simulink model "StandaloneDAQv07_R2014a"  (R2014a)
settings: Solver=FixedStepDiscrete  SolverMode=MultiTasking  StartTime=0.0  StopTime=inf  FixedStep=0.0005  RelTol=1e-3
values from neighbouring files (symbols this model uses):
  ANOMALY_INIT = 10    [DAQParams3_1ms_DDA.m]
  Calibration = getCalibrationParams_ATRIAS()    [DAQParams3_1ms_DDA.m]
  EnableFT = 0    [DAQParams3_1ms_DDA.m]
  EncoderAngleLimits = [60 240; 120 300; 60 240; 120 300; 60 240; 120 300; 60 240; 120 300; -30 30; -30 30; -inf inf; -inf inf; -inf inf; -inf inf; -30 30; -30 30; -inf inf; -90 90; -90 90]*pi/180    [DAQParams3_1ms_DDA.m]
  EncoderFiltSys = getDerivFilter(2, 5, 5, Ts)    [DAQParams3_1ms_DDA.m]
  EncoderThreshold = [5; 5; 5; 5; 5; 5; 5; 5; 5; 5; 250; 250; 250; 250; 5; 5; 5; 5; 5]*pi/180    [DAQParams3_1ms_DDA.m]
  IMUAngleLimits = [-180 180; -90 90; -90 90]*pi/180    [DAQParams3_1ms_DDA.m]
  IMUCommand = 70    [DAQParams3_1ms_DDA.m]
  IMUThreshold = 5*pi/180    (= 0.0872664625997)    [DAQParams3_1ms_DDA.m]
  MAX_ANOMALY = 30    [DAQParams3_1ms_DDA.m]
  MedullaCommand = 0    [DAQParams3_1ms_DDA.m]
  MicrostrainFiltSys = getDerivFilter(2, 5, 5, TsMicrostrain)    [DAQParams3_1ms_DDA.m]
  MODBUS_TIMEOUT = 0.02    [DAQParams3_1ms_DDA.m]
  ResetDAQ = 0    [DAQParams3_1ms_DDA.m]
  ResetYaw = 0    [DAQParams3_1ms_DDA.m]
  STREAMING_TIMEOUT = 0.1    [DAQParams3_1ms_DDA.m]
  TareFT = 0    [DAQParams3_1ms_DDA.m]
  Ts = 0.001    [DAQParams3_1ms_DDA.m]
  UseMicrostrainRate = 0    [DAQParams3_1ms_DDA.m]
undefined symbols (not defined in the file or in its folder): FTCalibration, GearOffset, IMUTorsoOffset, m_XR17D15x, standard
libraries: xpcethercatlib x167, speedgoatlib x13, dspswit3 x2, simulink x2, xpcseriallib x1, SpeedgoatModified x1
(part 4 of 4)

== matlab function StandaloneDAQv07_R2014a/SerialInterfaces/FTInterface/Subsystem/ComputeCalibratedTorques/ComputeCalibratedTorques ==
  data: Gauge input; FT output; Bias input; Cal input
function FT = fcn(Gauge, Bias, Cal)
    %#codegen
    FT = Cal.BasicMatrix * (Gauge - Bias);
    FT(1:3,:) = FT(1:3,:) / Cal.CountsPerForce;
    FT(4:6,:) = FT(4:6,:) / Cal.CountsPerTorque;
end

== stateflow chart StandaloneDAQv07_R2014a/EtherCATNetwork/EncoderFilters/CheckAndFilterEncoder/AnomalyDetection ==
  state Run
    state Nominal
      en, du:
      q_clean = q;
      q_last = q;
      dq_last = dq;
      Counter_last = Counter;
      ErrorCount = 0;
    state MissedPacket
      en, du:
      q_clean = q_last + dq_last*ANOMALY_DT;
      ErrorCount--;
    state Error
      en: dq_last = dq; //dq is delayed to prevent algebraic loops
      en, du:
      ErrorCount++;
      q_clean = q_last + ErrorCount*dq_last*ANOMALY_DT;
    (default) -> Nominal
    Nominal -> MissedPacket [order 1] : [0 && Counter == Counter_last]
    MissedPacket -> Nominal
    Nominal -> Error [order 2] : [check_error()]
    Error -> Nominal [order 2] : [!check_error()]
  state Init
    en, du:
    q_clean = q;
    q_last = q;
    dq_last = dq;
    ErrorCount = 0;
  (default) -> Init
  Init -> Run : [!Reset && after(ANOMALY_INIT, tick)]
  Run -> Init : [Reset]
  Error -> Init [order 1] : [ErrorCount>MAX_ANOMALY]
  data: err function_output boolean; q input size=1; dq input size=1; Counter input; q_clean output double size=1; ErrorCount output double; MAX_ANOMALY parameter double size=1; q_last local double size=1; dq_last local double size=1; ANOMALY_INIT parameter double size=1; q_limits input double size=2; Threshold input size=1; Reset input boolean size=1; ANOMALY_DT input double size=1; Counter_last local double size=1
  function err = check_error:
    | function err = check_error
    |     %#codegen
    |     err = (q<q_limits(1)) || (q>q_limits(2)) ...
    |         || (abs(q - q_clean) > (ErrorCount+1)*Threshold);
    | end

== matlab function StandaloneDAQv07_R2014a/EtherCATNetwork/EtherCATRobotMicrostrain/ConvertMotorVoltage ==
  data: adc_value input; motorVoltage output
function motorVoltage = convert(adc_value)
    %#codegen
    
    MOTOR_VOLTAGE_C_OFFSET    = 1300.0;
    MOTOR_VOLTAGE_V_CAL       = 60.2;
    MOTOR_VOLTAGE_C_CAL       = 3600.0;
    
    motorVoltage = (adc_value - MOTOR_VOLTAGE_C_OFFSET)*MOTOR_VOLTAGE_V_CAL/(MOTOR_VOLTAGE_C_CAL-MOTOR_VOLTAGE_C_OFFSET);
end

== matlab function StandaloneDAQv07_R2014a/EtherCATNetwork/EtherCATRobotMicrostrain/EncodeSwitches ==
  data: Switches input; LimitSwitchesEncoded output
function LimitSwitchesEncoded = EncodeSwitches(Switches)
    LimitSwitchesVec     = uint32(Switches);
    LimitSwitchesEncoded = double(EncodeSwitches(LimitSwitchesVec));
end

== matlab function StandaloneDAQv07_R2014a/SerialInterfaces/KVH/ComputeEulerAngles ==
  data: RkIn input; wk input; RCal input; Reset input; R0In input; ZYX output; dZYX output; Rk output; R0 output; YawRolloverIn input; YawRollover output
function [ZYX, dZYX, Rk, R0, YawRollover] = fcn(RkIn, wk, RCal, Reset, R0In, YawRolloverIn) %#codegen
    % Convert from IMU frame to robot frame and compute Euler angles. The
    % yaw angle is zeroed whenever (Reset) is true.
        
    if (Reset)
        % Compute the rotation matrix which zeroes the initial yaw
        qT0 = M_to_ZYX(RkIn*RCal);
        R0  = Rz(-qT0(1));
    else
        R0 = R0In;
    end
    
    % Transform from IMU to robot frame and zero initial yaw
    Rk = R0*RkIn*RCal;
    
    % Convert Rk to ZYX Euler angles
    ZYX = M_to_ZYX(Rk);
    
    % Unroll yaw
    YawRolloverCount = YawRolloverIn(1);
    PreviousYaw      = YawRolloverIn(2);
    CurrentYaw       = ZYX(1);
    YawRolloverCount = YawRolloverCount + getYawRollover(CurrentYaw, PreviousYaw);
    YawRollover      = [YawRolloverCount; CurrentYaw];
    ZYX(1)           = ZYX(1) + 2*pi*YawRolloverCount;
    
    % Compute Euler angle derivatives
    qzT = ZYX(1);
    qyT = ZYX(2);
    
    if cos(qyT)>1e-3
        dZYX = [0 -sin(qzT) cos(qzT)*cos(qyT); 0 cos(qzT) sin(qzT)*cos(qyT); 1 0 -sin(qyT)]\(R0*RkIn*wk);
    else
        dZYX = [0; 0; 0];
    end
end

function R = Rz(t)
    R = [cos(t) -sin(t) 0; sin(t) cos(t) 0; 0 0 1];
end

function Rollover = getYawRollover(CurrentYaw, PreviousYaw)
    % Determine if a rollover has occurred on yaw angle If a rollover is
    % detected, the output Rollover is either +1 or -1, depending on the
    % direction of the rollover.
  
    if (PreviousYaw>0 && CurrentYaw < (PreviousYaw-pi))
        Rollover = 1;
    elseif (PreviousYaw<0 && CurrentYaw > (PreviousYaw+pi))
        Rollover = -1;
    else
        Rollover = 0;
    end
end

== matlab function StandaloneDAQv07_R2014a/EtherCATNetwork/convert_mtr_current_to_pwm ==
  data: params input; u input; y output; Reset input
function y = convert_to_pwm(params,u,Reset)
%#codegen
%This function takes motor torque command inputs and outputs
%pwm commands (for the Medulla) in UMich convention

y = zeros(6,1);

if (Reset)
    return
end

%The inputs, which are commanded motor torques 
leg_motor_1R_torque_cmd = u(1);
leg_motor_2R_torque_cmd = u(2);
hip_motor_3R_torque_cmd = u(3);
leg_motor_1L_torque_cmd = u(4);
leg_motor_2L_torque_cmd = u(5);
hip_motor_3L_torque_cmd = u(6);

%Parameters determined experimentally at U Mich
UMich_LEFT_MOTOR_HIP_DIRECTION = params(1); %The direction for the left hip motor. (UMich convention)
UMich_RIGHT_MOTOR_HIP_DIRECTION = params(2); %The direction for the right hip motor. (UMich convention)

% The parameters, from http://code.google.com/p/atrias/source/browse/robot_definitions/
%From robot_invariant_defs.h
MTR_MAX_COUNT = params(3); %The maximum commanded amplifier value. This is the maximum value sent to the Medullas for the amplifier command.
%From biped2_variant_defs.h
MTR_MAX_TORQUE = params(4); %Maximum motor torque for scaling
MTR_HIP_MAX_TORQUE = params(5); %Maximum hip motor torque for scaling
%From leg3_definitions.h (corresponds to our left leg)
%(Note that A=shin and B=thigh for OSU convention)
LEG3_MOTOR_A_DIRECTION = params(6);
LEG3_MOTOR_B_DIRECTION = params(7);
%From leg4_definitions.h (corresponds to our right leg)
%(Note that A=shin and B=thigh for OSU convention)
LEG4_MOTOR_A_DIRECTION = params(8);
LEG4_MOTOR_B_DIRECTION = params(9);

leg_torque_to_pwm = MTR_MAX_COUNT/MTR_MAX_TORQUE;
hip_torque_to_pwm = MTR_MAX_COUNT/MTR_HIP_MAX_TORQUE;

%Convert leg_motor_1L_torque_cmd
leg_motor_1L_direction = LEG3_MOTOR_A_DIRECTION;
y(1) = motor_torque_to_pwm(leg_motor_1L_direction,leg_torque_to_pwm,leg_motor_1L_torque_cmd);

%Convert leg_motor_2L_torque_cmd
leg_motor_2L_direction = LEG3_MOTOR_B_DIRECTION;
y(2) = motor_torque_to_pwm(leg_motor_2L_direction,leg_torque_to_pwm,leg_motor_2L_torque_cmd);

%Convert leg_motor_1R_torque_cmd
leg_motor_1R_direction = LEG4_MOTOR_A_DIRECTION;
y(3) = motor_torque_to_pwm(leg_motor_1R_direction,leg_torque_to_pwm,leg_motor_1R_torque_cmd);

%Convert leg_motor_2R_torque_cmd
leg_motor_2R_direction = LEG4_MOTOR_B_DIRECTION;
y(4) = motor_torque_to_pwm(leg_motor_2R_direction,leg_torque_to_pwm,leg_motor_2R_torque_cmd);

%Convert hip_motor_3R_torque_cmd
hip_motor_3R_direction = UMich_RIGHT_MOTOR_HIP_DIRECTION; %Verified experimentally
y(5) = motor_torque_to_pwm(hip_motor_3R_direction,hip_torque_to_pwm,hip_motor_3R_torque_cmd);

%Convert hip_motor_3L_torque_cmd
hip_motor_3L_direction = UMich_LEFT_MOTOR_HIP_DIRECTION; %Verified experimentally
y(6) = motor_torque_to_pwm(hip_motor_3L_direction,hip_torque_to_pwm,hip_motor_3L_torque_cmd);

end

function motor_pwm = motor_torque_to_pwm(motor_direction,torque_to_pwm_const,motor_torque_cmd)
   motor_pwm = motor_direction*torque_to_pwm_const*motor_torque_cmd;
end
